simulink model "anomaly_stateflow"  (R2025b)
settings: Solver=VariableStepAuto  StartTime=0.0  StopTime=10.0  RelTol=1e-3
settings Model: Creator=strog  LastModifiedBy=strog

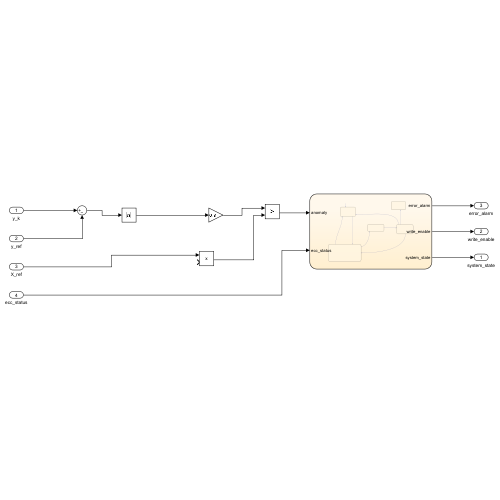
[thumbnail: Simulink's stored preview of the top-level diagram]
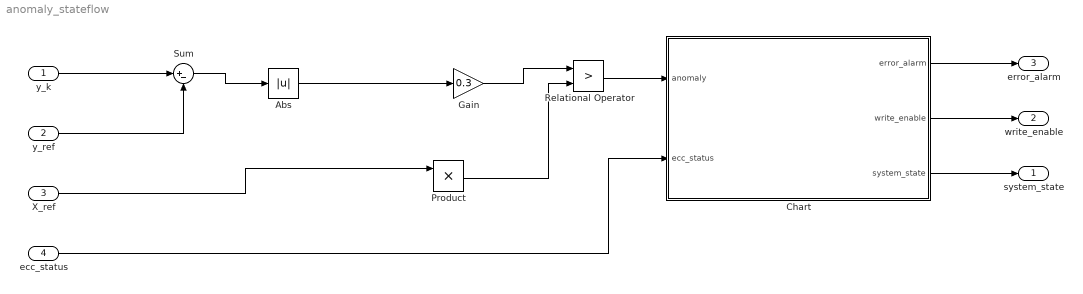
== system anomaly_stateflow ==
  y_k : Inport
  y_ref : Inport  Port=2
  X_ref : Inport  Port=3
  ecc_status : Inport  Port=4
  Abs : Abs  SaturateOnIntegerOverflow=off
  Chart : Stateflow chart  TreatAsAtomicUnit=on
  Gain : Gain  Gain=0.3
  Product : Product
  Relational Operator : RelationalOperator  Operator=>  OutDataTypeStr=boolean  RndMeth=Simplest  InputSameDT=off
  Sum : Sum  Inputs=|+-
  system_state : Outport
  write_enable : Outport  Port=2
  error_alarm : Outport  Port=3
  wires:
  Chart/2(write_enable) -> write_enable/1
  y_ref/1 -> Sum/2
  Product/1 -> Relational Operator/2
  Gain/1 -> Relational Operator/1
  Sum/1 -> Abs/1
  y_k/1 -> Sum/1
  X_ref/1 -> Product/1
  Abs/1 -> Gain/1
  Chart/1(error_alarm) -> error_alarm/1
  Chart/3(system_state) -> system_state/1
  Relational Operator/1 -> Chart/1(anomaly)
  ecc_status/1 -> Chart/2(ecc_status)

== stateflow chart anomaly_stateflow/Chart ==
  state Error
    entry:
    write_enable = false;
    error_alarm = true;
    system_state = 5;
  state Normal
    entry:
    write_enable = false;
    error_alarm = false;
    system_state = 1;
  state Snapshot
    entry:
    write_enable = true;
    system_state = 3;
  state RetryECC
    entry:
    write_enable = false;
    system_state = 4;
  state Alarm
    entry:
    anomaly_counter = 0;
    during:
    if anomaly
    anomaly_counter = anomaly_counter + 1;
    else
    anomaly_counter = 0;
    end
    system_state=2;
  (default) -> Normal
  RetryECC -> Error [order 2] : [ecc_status==2]
  RetryECC -> Normal [order 3] : [ecc_status == 0 | (ecc_status == 1 & ~anomaly)]
  Alarm -> Normal [order 2] : [~anomaly]
  Normal -> Alarm : [anomaly]
  Snapshot -> RetryECC
  Alarm -> Snapshot [order 1] : [anomaly_counter>=3]
  RetryECC -> Alarm [order 1] : [ecc_status ==1 & anomaly]
  data: anomaly input; ecc_status input; error_alarm output; write_enable output; anomaly_counter local; system_state output
